simulink model "feedbacklinearization"  (R2013b)
settings: Solver=ode45  StartTime=0.0  StopTime=10  RelTol=1e-3
libraries: simulink_extras x2
settings Model: Creator=Maksimus  LastModifiedBy=Maksimus

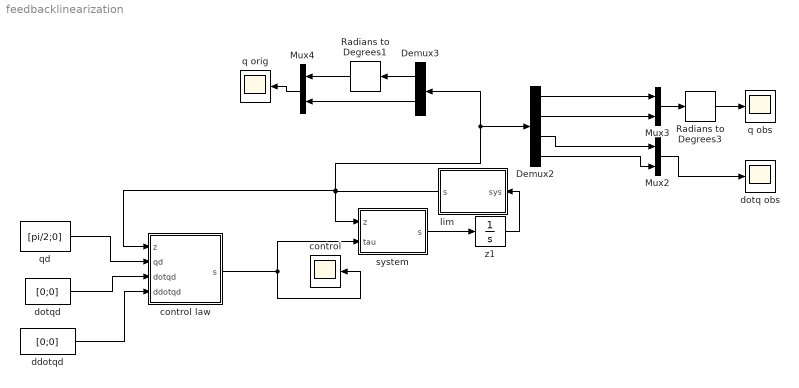
== system feedbacklinearization ==
  Demux2 : Demux
  Demux3 : Demux  Outputs=2
  Mux2 : Mux  Inputs=2
  Mux3 : Mux  Inputs=2
  Mux4 : Mux  Inputs=2
  Radians to Degrees1 : simulink_extras/Transformations/Radians to Degrees
  Radians to Degrees3 : simulink_extras/Transformations/Radians to Degrees
  control : Scope
      settings: TimeRange=5  YMin=4e+06  YMax=1.25e+07  SaveName=CFEED
  control law : MATLAB Function  TreatAsAtomicUnit=on
  ddotqd : Constant  Value=[0;0]
  dotq obs : Scope
      settings: YMin=-5.5e+06  YMax=4e+06
  dotqd : Constant  Value=[0;0]
  lim : MATLAB Function  TreatAsAtomicUnit=on
  q obs : Scope
      settings: YMin=-350  YMax=350
  q orig : Scope
      settings: YMin=-350  YMax=350  SaveName=FEED
  qd : Constant  Value=[pi/2;0]
  system : MATLAB Function  TreatAsAtomicUnit=on
  z1 : Integrator  InitialCondition=[0;0;0;0]  IgnoreLimit=on
  wires:
  system/1(s) -> z1/1
  Demux2/1 -> Mux3/1
  Mux3/1 -> Radians to Degrees3/1
  Radians to Degrees3/1 -> q obs/1
  Demux2/4 -> Mux2/2
  Demux2/3 -> Mux2/1
  Demux2/2 -> Mux3/2
  control law/1(s) -> system/2(tau), control/1
  Mux2/1 -> dotq obs/1
  qd/1 -> control law/2(qd)
  dotqd/1 -> control law/3(dotqd)
  ddotqd/1 -> control law/4(ddotqd)
  z1/1 -> lim/1(sys)
  Demux3/1 -> Radians to Degrees1/1
  Demux3/2 -> Mux4/2
  Mux4/1 -> q orig/1
  lim/1(s) -> Demux2/1, Demux3/1, control law/1(z), system/1(z)
  Radians to Degrees1/1 -> Mux4/1

== matlab function feedbacklinearization/system ==
  data: z input; s output; tau input
function s = fcn(z,tau)
%global linA linB linConst
%s = linA * z + linB * u + linConst;
m1 = 1; m2 = 1;
lc1 = 0.5; lc2 = 0.5;
I1 = 0.12; I2 = 0.12;
l1 = 1; l2 = 1;
g=10;

m = [m1;m2];
lc = [lc1;lc2];
I = [I1;I2];
l = [l1;l2];
dotq = z(3:4);
q = z(1:2);
theta = [m(1)*lc(1)^2 + m(2)*l(1)^2 + I(1); m(2) * lc(2)^2 + I(2); m(2)*l(1)*lc(2); m(1)*lc(1) + m(2)*l(1); m(2)*lc(2)]; 

H = [theta(1) + theta(2) + 2 * theta(3)*cos(q(2)), theta(2) + theta(3) * cos(q(2));
    theta(2) + theta(3) * cos(q(2)), theta(2)]; %is symmetrie, positive definite for all q

%H(q) - 2C(q, dotq) is a skew-syrnmetric matrix

C = [-theta(3) * sin(q(2)) * dotq(2), -theta(3) * sin(q(2)) * dotq(2) - theta(3) * sin(q(2)) * dotq(1);
    theta(3) * sin(q(2)) * dotq(1), 0];

G = [ theta(4) * g * cos(q(1)) + theta(5) * g * cos(q(1) + q(2)); theta(5) * g * cos(q(1) + q(2))]; %nonhorizontal robotarm
%G = [0;0];

InvH = H^(-1);
InvHC = InvH * C;
InvHG = InvH * G;
tmpsys = - InvHC * dotq - InvHG + InvH*tau;
sys = [dotq;tmpsys];

s = sys;

== matlab function feedbacklinearization/control law ==
  data: z input; qd input; s output; dotqd input; ddotqd input
function s = fcn(z,qd, dotqd, ddotqd)
%задаем систему
m1 = 1; m2 = 1;
lc1 = 0.5; lc2 = 0.5;
I1 = 0.12; I2 = 0.12;
l1 = 1; l2 = 1;
g=10;
m = [m1;m2];
lc = [lc1;lc2];
I = [I1;I2];
l = [l1;l2];
q =z(1:2);
dotq =z(3:4);

theta = [m(1)*lc(1)^2 + m(2)*l(1)^2 + I(1); m(2) * lc(2)^2 + I(2); m(2)*l(1)*lc(2); m(1)*lc(1) + m(2)*l(1); m(2)*lc(2)]; 

H = [theta(1) + theta(2) + 2 * theta(3)*cos(q(2)), theta(2) + theta(3) * cos(q(2));
    theta(2) + theta(3) * cos(q(2)), theta(2)]; 

C = [-theta(3) * sin(q(2)) * dotq(2), -theta(3) * sin(q(2)) * dotq(2) - theta(3) * sin(q(2)) * dotq(1);
    theta(3) * sin(q(2)) * dotq(1), 0];

G = [ theta(4) * g * cos(q(1)) + theta(5) * g * cos(q(1) + q(2)); theta(5) * g * cos(q(1) + q(2))]; %nonhorizontal robotarm
%конец задания системы
%G = [0;0];

lambda = 5;
v = ddotqd - 2*lambda * (dotq - dotqd) - lambda^2 * (q - qd);
InvH = H^(-1);
%InvHC = InvH * C;
%InvHG = InvH * G;
sys = H * v + C * dotq + G;

for i =1:length(sys)
    if abs(sys(i))>50
        if sys(i) > 50
            sys(i) = 50;
        else
            sys(i) = -50;
        end
    end
end

s = sys;

== matlab function feedbacklinearization/lim ==
  data: sys input; s output
function s = fcn(sys)

ogr = [2*pi;pi;5;5];
for i =1:length(sys)
    if i == 1
        if sys(i)> ogr(i)
            sys(i) = ogr(i);
        elseif sys(i) < 0 
            sys(i) = 0;
        end
    elseif abs(sys(i))>ogr(i)
        if sys(i) > ogr(i)
            sys(i) = ogr(i);
        else
            sys(i) = -ogr(i);
        end
    end
end
s = sys;
